simulink model "Courant"  (R2021a)
settings: Solver=VariableStepAuto  StartTime=0.0  StopTime=0.2  FixedStep=0.001  RelTol=1e-3
values from neighbouring files (symbols this model uses):
  L = 0.115    [Courant_matlab.m]
  R = 3.6    [Courant_matlab.m]
settings Model: Creator=dupa1607  LastModifiedBy=dupa1607
settings SolverCC: AlgebraicLoopSolver=TrustRegion
settings DebuggingCC: SFMachineParentedDataDiag=warning

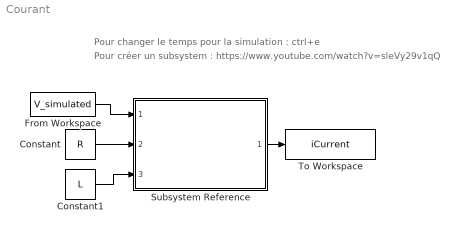
== system Courant ==
  note: Pour créer un subsystem : https://www.youtube.com/watch?v=sleVy29v1qQ
  note: Pour changer le temps pour la simulation : ctrl+e
  Constant : Constant  Value=R
  Constant1 : Constant  Value=L
  From Workspace : FromWorkspace  VariableName=V_simulated
  Subsystem Reference : Subsystem  ReferencedSubsystem=subsys_courant
  To Workspace : ToWorkspace  VariableName=iCurrent  SaveFormat=Timeseries  SampleTime=-1
  wires:
  Subsystem Reference/1 -> To Workspace/1
  From Workspace/1 -> Subsystem Reference/1
  Constant/1 -> Subsystem Reference/2
  Constant1/1 -> Subsystem Reference/3
